simulink model "FM_Simulink"  (R2017b)
settings: Solver=VariableStepAuto  StartTime=0.0  StopTime=10.0  RelTol=1e-3
libraries: rtlsdr_book_library x4, dspmlti4 x2, dspsnks4 x1, sdrrlib x1
settings Model: Creator=Nasa  LastModifiedBy=Nasa

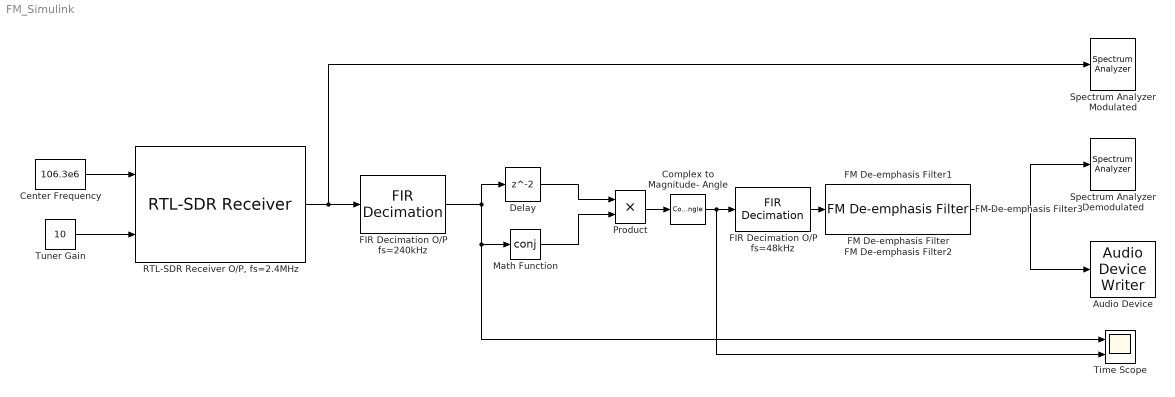
== system FM_Simulink ==
  "Audio Device " : dspsnks4/Audio Device Writer  Driver=DirectSound  Device=Speaker/Headphone (Realtek High Definition Audio)  InheritSampleRate=on  SampleRate=44100  BitDepth=16-bit integer  BufferSize=4096  NumBuffers=10  DefaultOutputChannelMapping=on  OutputChannelMapping=1:2  OutputNumUnderrunSamples=off  DriverIdx=1  DeviceWarnFlag=''
  Center Frequency : Constant  Value=106.3e6
  Complex to Magnitude- Angle : ComplexToMagnitudeAngle  Output=Angle
  Delay : Delay  InputProcessing=Columns as channels (frame based)
  FIR Decimation O/P fs=240kHz : dspmlti4/FIR Decimation  FilterSource=Dialog parameters  h=firpm(50,[0 120e3 240e3 (2.4e6/2)]/(2.6e6/2),[1 1 0 0],[1 1],20)  D=10  filtStruct=Direct form  FilterObject=FDECIM  InputProcessing=Columns as channels (frame based)  framing=Allow multirate processing  inputOffset=0  outputBufInitCond=0  roundingMode=Floor  overflowMode=off  firstCoeffDataTypeStr=Inherit: Same word length as input  firstCoeffMin=[]  firstCoeffMax=[]  firstCoeffLastDataTypeStr=Inherit: Same word length as input  outputDataTypeStr=Inherit: Same as accumulator  outputMin=[]  outputMax=[]  outputLastDataTypeStr=Inherit: Same as accumulator
  FIR Decimation O/P fs=48kHz : dspmlti4/FIR Decimation  FilterSource=Dialog parameters  h=firpm(100,[0 15e3 20e3 (240e3/2)]/(240e3/2),[1 1 0 0],[1 1],20)  D=5  filtStruct=Direct form  FilterObject=FDECIM  InputProcessing=Columns as channels (frame based)  framing=Allow multirate processing  inputOffset=0  outputBufInitCond=0  roundingMode=Floor  overflowMode=off  firstCoeffDataTypeStr=Inherit: Same word length as input  firstCoeffMin=[]  firstCoeffMax=[]  firstCoeffLastDataTypeStr=Inherit: Same word length as input  outputDataTypeStr=Inherit: Same as accumulator  outputMin=[]  outputMax=[]  outputLastDataTypeStr=Inherit: Same as accumulator
  FM De-emphasis Filter{,1..3} (4 alike) : rtlsdr_book_library/FM Demod Tools/FM De-emphasis Filter  region=Europe, Asia  fs=48e3
      settings: SourceProductName=RTL-SDR Book Library
  Math Function : Math  Operator=conj  SaturateOnIntegerOverflow=on
  Product : Product  Inputs=**
  "RTL-SDR Receiver O/P, fs=2.4MHz" : sdrrlib/RTL-SDR Receiver  SourceLibraryInfo="This block requires <a href=\"http://www.mathworks.com/hardware-support/rtl-sdr.html\">Communications System Toolbox Support Package for RTL-SDR Radio</a>"  IPAddress=0  CenterFrequencySource=Input port  CenterFrequency=102.5e6  GainSource=Input port  Gain=0  ADCRate=2.4e6  FrequencyCorrection=0  LostSamplesOutputPort=off  LatencyOutputPort=off  OutputDataType=single  FrameLength=4096  EnableBurstMode=off  NumFramesInBurst=20  sobjType=sdrr.internal.SDRRTLReceiverSL  dataUDPPort=-1  ctrlUDPPort=-1  subDeviceList=nosubdev  sdrBlockType=SDRBlockTypeSLT.SDRRxBlock  requester=UNUSED_BY_SFCN  sdrExecutionMode=SDRExecutionModeSLT.ExecModeHW  BypassUserLogic=off  DecimatorSelect=DDC decimator  SourceSelect=RF data  SineAmplitude=16000  EnableInternalClock=off  BypassIQBalance=off  IFBandwidth=40e6  ADCRateSource=Dialog  IntermediateFrequency=0  DecimationFactorSource=Dialog  DecimationFactor=512  RFFrequencyIsTunable=logical(1)  SampleTime=(4096)/(2.4e6)  IFBandwidthSource=Dialog  SineFrequency=30000  BypassDCBlockingFilter=off  IntermediateFrequencySource=Dialog  IQBalanceCoefficients=64  SkipAllHardwareResetAndInitialization=off  EnableIQCalibrationTable=on  CacheIQCalibrationTable=off  EnableOffsetTuning=off  EnableRTLAGC=off  EnableTestMode=off  EnableTunerAGC=on  FrequencyCorrectionSource=Dialog  NumMLBuffers=128  NumUSBBuffers=16  RTLCrystalFrequency=28800000  TunerCrystalFrequency=28800000
      settings: SourceProductName=Communications System Toolbox Support Package for RTL-SDR Radio  SourceProductBaseCode=RTLSDR
  Spectrum Analyzer Demodulated : SpectrumAnalyzer
  Spectrum Analyzer Modulated : SpectrumAnalyzer
  Time Scope : Scope  NumInputPorts=2
  Tuner Gain : Constant  Value=10
  wires:
  "RTL-SDR Receiver O/P, fs=2.4MHz"/1 -> Spectrum Analyzer Modulated/1, FIR Decimation O/P fs=240kHz/1
  Center Frequency/1 -> "RTL-SDR Receiver O/P, fs=2.4MHz"/1
  Tuner Gain/1 -> "RTL-SDR Receiver O/P, fs=2.4MHz"/2
  Delay/1 -> Product/1
  Math Function/1 -> Product/2
  Product/1 -> Complex to Magnitude- Angle/1
  FIR Decimation O/P fs=240kHz/1 -> Time Scope/1, Math Function/1, Delay/1
  Complex to Magnitude- Angle/1 -> Time Scope/2, FIR Decimation O/P fs=48kHz/1
  FIR Decimation O/P fs=48kHz/1 -> FM De-emphasis Filter/1
  FM De-emphasis Filter/1 -> Spectrum Analyzer Demodulated/1, "Audio Device "/1
